simulink model "soojen"  (R2017b)
settings: Solver=ode45  StartTime=0.0  StopTime=11000.0  RelTol=1e-3  EnableMultiTasking=on
values from neighbouring files (symbols this model uses):
  A = [2.2 4.3 ... (first row only)    [YL_D_12.m]    (also in YL_E_9.m = [0.3479 0.6521 0.6521 0.3479]; analuus.m = [1 0;2 -2], B=[-2; -1], K=[0 0]; kodutoo1.m = [ 0 0 1 0;  0 0 0 1;  0 m*g/M -D/M 0;  0 -(M+m)*g/(M*L) D/(M)
  c = inv(A)*B'    [Arvutusmeetodid11_1.m]    (also in Arvutusmeetodid11_2.m = inv(A)*b'; Arvutusmeetodid12_3.m; Yl_B_6.m = d; Yl_B_6_2.m = d)
  m = 1.e-9    (= 1e-09)    [lorentz.m]
undefined symbols (not defined in the file or in its folder): Ak, U, Uk
settings Model: Creator=andres  LastModifiedBy=Andres
settings DataIOCC: LimitDataPoints=on  SaveFormat=Array  SignalLoggingSaveFormat=ModelDataLogs
settings OptimizationCC: ExpressionDepthLimit=2147483647  InitFltsAndDblsToZero=on  LifeSpan=inf
settings DebuggingCC: SaveWithParameterizedLinksMsg=none  UnderspecifiedInitializationDetection=Classic  MergeDetectMultiDrivingBlocksExec=none  SolverPrmCheckMsg=warning  FcnCallInpInsideContextMsg=warning  StateNameClashWarn=warning  SFUnexpectedBacktrackingDiag=warning  SFNoUnconditionalDefaultTransitionDiag=warning  SFExecutionAtInitializationDiag=none
settings HardwareCC: ProdBitPerPointer=32  ProdBitPerSizeT=32  ProdBitPerPtrDiffT=32  ProdLargestAtomicFloat=None  ProdIntDivRoundTo=Undefined  ProdEndianess=Unspecified  ProdWordSize=32  ProdHWDeviceType=32-bit Generic
settings ModelReferenceCC: PropagateSignalLabelsOutOfModel=off
settings CodeAppCC: StateflowObjectComments=on
settings GRTTargetCC: TargetFcnLib=ansi_tfl_tmw.mat  TargetLangStandard=C89/C90 (ANSI)  CombineOutputUpdateFcns=off  GRTInterface=on
settings ConfigComp: CovMetricSettings=dw  CovHtmlReporting=on  CovSaveCumulativeToWorkspaceVar=on  CovSaveSingleToWorkspaceVar=on  CovExternalEMLEnable=off

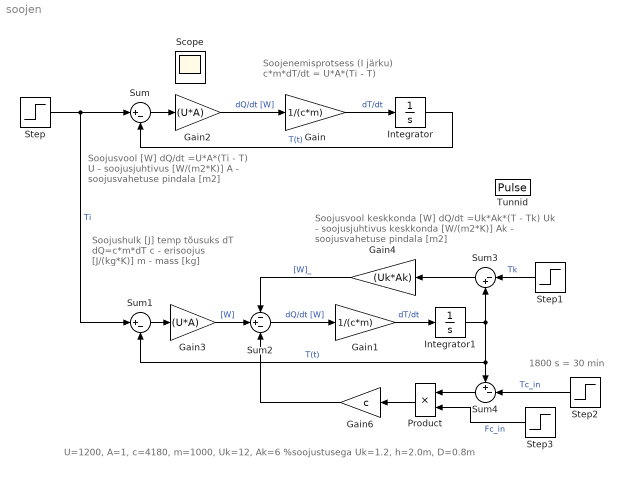
== system soojen ==
  note: Soojusvool [W]
      | dQ/dt =U*A*(Ti - T)
      | U - soojusjuhtivus [W/(m2*K)]
      | A - soojusvahetuse pindala [m2]
  note: Soojushulk [J] temp tõusuks dT
      | dQ=c*m*dT
      | c - erisoojus [J/(kg*K)]
      | m - mass [kg]
  note: Soojenemisprotsess (I järku)
      | c*m*dT/dt = U*A*(Ti - T)
  note: 1800 s = 30 min
  note: Soojusvool keskkonda [W] dQ/dt =Uk*Ak*(T - Tk)
      | Uk - soojusjuhtivus keskkonda [W/(m2*K)]
      | Ak - soojusvahetuse pindala [m2]
  note: U=1200, A=1, c=4180, m=1000, Uk=12, Ak=6 %soojustusega Uk=1.2, h=2.0m, D=0.8m
  Gain : Gain  Gain=1/(c*m)
  Gain1 : Gain  Gain=1/(c*m)
  Gain2 : Gain  Gain=(U*A)
  Gain3 : Gain  Gain=(U*A)
  Gain4 : Gain  Gain=(Uk*Ak)
  Gain6 : Gain  Gain=c
  Integrator : Integrator  InitialCondition=15
  Integrator1 : Integrator  InitialCondition=15
  Product : Product  RndMeth=Zero
  Step : Step  Time=0  After=60  SampleTime=0
  Step1 : Step  Time=0  After=15  SampleTime=0
  Step2 : Step  Time=0  After=15  SampleTime=0
  Step3 : Step  Time=1800  After=0.2  SampleTime=0
  Sum : Sum  Inputs=|+-
  Sum1 : Sum  Inputs=|+-
  Sum2 : Sum  Inputs=-+-
  Sum3 : Sum  Inputs=|-+
  Sum4 : Sum  Inputs=+-|
  Tunnid : DiscretePulseGenerator  PulseType=Time based  Amplitude=60  Period=3600
  Scope : Scope
  wires:
  Step/1 -> Sum/1, Sum1/1  "Ti"
  Sum/1 -> Gain2/1
  Gain/1 -> Integrator/1  "dT/dt"
  Integrator/1 -> Sum/2  "T(t)"
  Gain2/1 -> Gain/1  "dQ/dt [W]"
  Sum1/1 -> Gain3/1
  Gain1/1 -> Integrator1/1  "dT/dt"
  Integrator1/1 -> Sum3/2, Sum1/2, Sum4/1  "T(t)"
  Gain3/1 -> Sum2/2  "[W]"
  Sum2/1 -> Gain1/1  "dQ/dt [W]"
  Gain4/1 -> Sum2/1  "[W]_"
  Step1/1 -> Sum3/1  "Tk"
  Sum3/1 -> Gain4/1
  Gain6/1 -> Sum2/3
  Step2/1 -> Sum4/2  "Tc_in"
  Product/1 -> Gain6/1
  Sum4/1 -> Product/1
  Step3/1 -> Product/2  "Fc_in"
